simulink model "dsp48e_bram_vacc_blk"  (R2019a)
settings: Solver=VariableStepAuto  StartTime=0.0  StopTime=100  RelTol=1e-3
libraries: xbsIndex_r4 x1
settings Model: Creator=mybur  LastModifiedBy=mybur

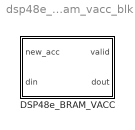
== system dsp48e_bram_vacc_blk ==
  DSP48e_BRAM_VACC : Subsystem  mask{vector_length=6, arith_type=off, bin_pt_out=0, n_bits_out=18, dsp_version=1}
      mask prompts: vector_length "Vector length:"; arith_type "Signed output?"; bin_pt_out "Binary point (output)"; n_bits_out "Bit width (output)"; dsp_version "DSP48e version:"
      mask init:
      | Simulink.Block.eval([gcb, '/dsp48e_bram_vacc']);
      mask TypeOptions dsp_version: 1 | 2
      mask DialogControl DescTextVar Prompt: A vector accumulator modeled after a shift register.  It outputs its previous accumulated vector after a new_acc pulse is received.  Based on the simple_bram_vacc block, this version replaces the adder and mux with a single DSP48E block, allowing high-speed compilation.  Output bit width cannot exceed 32. Output binary point matches the input.

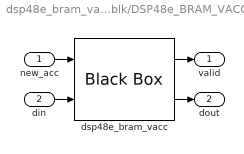
== system dsp48e_bram_vacc_blk/DSP48e_BRAM_VACC ==
  new_acc : Inport
  din : Inport  Port=2
  dsp48e_bram_vacc : xbsIndex_r4/Black Box  init_code=dsp48e_bram_vacc_config  sim_method=ISE Simulator  verbose=off  block_type=blackbox2
  valid : Outport
  dout : Outport  Port=2
  wires:
  dsp48e_bram_vacc/2 -> dout/1
  dsp48e_bram_vacc/1 -> valid/1
  din/1 -> dsp48e_bram_vacc/2
  new_acc/1 -> dsp48e_bram_vacc/1
